simulink model "damping"  (R2018b)
settings: Solver=VariableStepAuto  StartTime=0.0  StopTime=tsim  RelTol=1e-3
undefined symbols (not defined in the file or in its folder): tetherb
libraries: vrlib x1
settings Model: Creator=Erin B  LastModifiedBy=Erin B

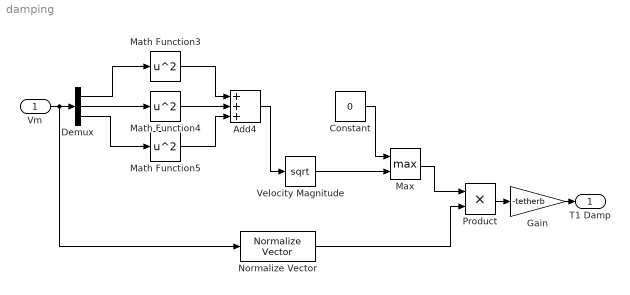
== system damping ==
  Vm : Inport  PortDimensions=3
  Add4 : Sum  Inputs=+++
  Constant : Constant  Value=0
  Demux : Demux  Outputs=3
  Gain : Gain  Gain=-tetherb
  Math Function3 : Math  Operator=square  SaturateOnIntegerOverflow=on
  Math Function4 : Math  Operator=square  SaturateOnIntegerOverflow=on
  Math Function5 : Math  Operator=square  SaturateOnIntegerOverflow=on
  Max : MinMax  Function=max  Inputs=2
  Normalize Vector : vrlib/Utilities/Normalize Vector  maxzero=0
      settings: SourceProductName=Simulink 3D Animation  SourceProductBaseCode=VR
  Product : Product
  Velocity Magnitude : Sqrt  SaturateOnIntegerOverflow=on
  T1 Damp : Outport
  wires:
  Vm/1 -> Normalize Vector/1, Demux/1
  Demux/3 -> Math Function5/1
  Math Function5/1 -> Add4/3
  Math Function3/1 -> Add4/1
  Math Function4/1 -> Add4/2
  Add4/1 -> Velocity Magnitude/1
  Demux/1 -> Math Function3/1
  Demux/2 -> Math Function4/1
  Normalize Vector/1 -> Product/2
  Velocity Magnitude/1 -> Max/2
  Constant/1 -> Max/1
  Max/1 -> Product/1
  Product/1 -> Gain/1
  Gain/1 -> T1 Damp/1
